simulink model "EncoderOffsetCalibrationF28069mLaunchPad"  (R2025b)
settings: Solver=FixedStepDiscrete  StartTime=0.0  StopTime=2  FixedStep=Ts  RelTol=1e-3  EnableMultiTasking=on
InitFcn:
  | OffsetCalibrationCallback;
  | motor.QEPSlits   = eval(get_param([bdroot '/Offset Calculation/Parameters/QEP Slits'], 'Value'));
  | target = mcb.getProcessorParameters('F28069M',PWM_frequency);
values from neighbouring files (symbols this model uses):
  PWM_frequency = eval(get_param([bdroot '/Open Loop Control/Parameters/PWM Frequency'], 'Value'))    [OpenloopMotorControlCallback.m]    (also in setup_offset_calculations.m = 20000)
  Ts = T_pwm    [OpenloopMotorControlCallback.m]    (also in setup_offset_calculations.m = 5e-05)
undefined symbols (not defined in the file or in its folder): bit, Down, GPTRIP1SEL, GPTRIP2SEL, TZ1, TZ2, Up
libraries: c2802xlib x4, simulink x3, mcbcontrolslib x3, c280xlib x3, svdschedulerlib x2, c2806xlib x2, mcbpositiondecoderlib x2, mcbeeMathTransformLib x1

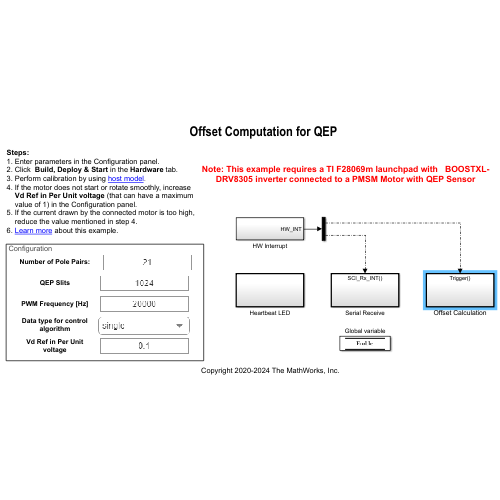
[thumbnail: Simulink's stored preview of the top-level diagram]
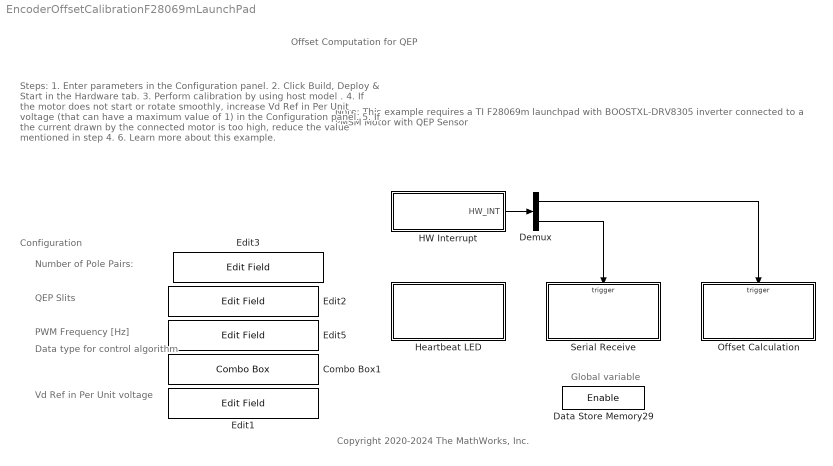
== system EncoderOffsetCalibrationF28069mLaunchPad ==
  note: Global variable
  note: Offset Computation for QEP
  note: Copyright 2020-2024 The MathWorks, Inc.
  note: QEP Slits
  note: PWM Frequency [Hz]
  note: Configuration
  note: Number of Pole Pairs:
  note: Data type for control algorithm
  note: Note: This example requires a TI F28069m launchpad with BOOSTXL-DRV8305 inverter connected to a PMSM Motor with QEP Sensor
  note: Steps:
      | 1. Enter parameters in the Configuration panel.
      | 2. Click Build, Deploy & Start in the Hardware tab.
      | 3. Perform calibration by using host model .
      | 4. If the motor does not start or rotate smoothly, increase
      | Vd Ref in Per Unit voltage (that can have a maximum
      | value of 1) in the Configuration panel.
      | 5. If the current drawn by the connected motor is too high,
      | reduce the value mentioned in step 4.
      | 6. Learn more about this example.
  note: Vd Ref in Per Unit voltage
  Combo Box1 : ComboBox  LabelPosition=Hide  SelectedLabel=single
  Data Store Memory29 : DataStoreMemory  DataStoreName=Enable  ReadBeforeWriteMsg=warning  WriteAfterWriteMsg=warning  WriteAfterReadMsg=warning  ShowAdditionalParam=off  OutDataTypeStr=boolean
  Demux : Demux  Outputs=2
  Edit{1..3,5} (4 alike) : EditField  LabelPosition=Hide  ShowInitialText=on  Alignment=Center
  HW Interrupt : Subsystem
  Heartbeat LED : Subsystem  TreatAsAtomicUnit=on
  Offset Calculation : Subsystem
  Serial Receive : Subsystem  SystemSampleTime=1e-3
  wires:
  HW Interrupt/1(HW_INT) -> Demux/1
  Demux/2 -> Serial Receive/Trigger
  Demux/1 -> Offset Calculation/Trigger

== system EncoderOffsetCalibrationF28069mLaunchPad/HW Interrupt ==
  HWI_ADCINT1 : svdschedulerlib/Hardware Interrupt v2  ISRGroup=ADC - Analog to Digital Converter  ISRName=ADCA1_INT  ISRNumber=32  NumEventsToServe=1  EventsList={'on','EOC event','1';'off','Overflow event','2';'off','Custom event','3'}  SelectedEvents={'event1'}  TaskPriority=30  DisablePreemption=off  ClearInterruptFlagsAtEndOfEvent=on  InterruptDefinitionFile=$(TARGET_ROOT)/registry/interrupts/F2837xS_interrupts.xml  HardwareBoard=F2837x  EnableSimPort=off
  HWI_SCIRXINTA : svdschedulerlib/Hardware Interrupt v2  ISRGroup=ADC - Analog to Digital Converter  ISRName=ADCA1_INT  ISRNumber=32  NumEventsToServe=1  EventsList={'on','EOC event','1';'off','Overflow event','2';'off','Custom event','3'}  SelectedEvents={'event1'}  TaskPriority=50  DisablePreemption=on  ClearInterruptFlagsAtEndOfEvent=on  InterruptDefinitionFile=$(TARGET_ROOT)/registry/interrupts/F2837xS_interrupts.xml  HardwareBoard=F2837x  EnableSimPort=off
  Mux : Mux  Inputs=2
  HW_INT : Outport
  wires:
  Mux/1 -> HW_INT/1
  HWI_ADCINT1/1 -> Mux/1
  HWI_SCIRXINTA/1 -> Mux/2

== system EncoderOffsetCalibrationF28069mLaunchPad/Heartbeat LED ==
  Digital Output1 : c2806xlib/Digital Output  GPIO_Number=GPIO32~GPIO39  GPIO_Bit0=off  GPIO_BIT0_Toggle=off  GPIO_Bit1=off  GPIO_BIT1_Toggle=off  GPIO_Bit2=on  GPIO_BIT2_Toggle=on  GPIO_Bit3=off  GPIO_BIT3_Toggle=off  GPIO_Bit4=off  GPIO_BIT4_Toggle=off  GPIO_Bit5=off  GPIO_BIT5_Toggle=off  GPIO_Bit6=off  GPIO_BIT6_Toggle=off  GPIO_Bit7=off  GPIO_BIT7_Toggle=off
  LED 1 Hz : Constant  OutDataTypeStr=uint16  SampleTime=0.5
  wires:
  LED 1 Hz/1 -> Digital Output1/1

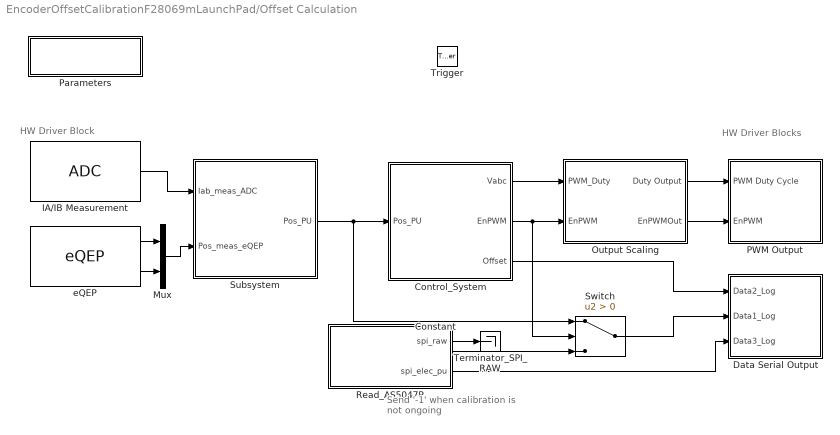
== system EncoderOffsetCalibrationF28069mLaunchPad/Offset Calculation ==
  note: HW Driver Blocks
  note: HW Driver Block
  note: Send '-1' when calibration is not ongoing
  Trigger : TriggerPort  TriggerType=function-call  VariantControl=Variant  PortDimensions=1
  Constant : Constant  Value=-1  OutDataTypeStr=dataType
  Control_System : Subsystem
  Data Serial Output : Subsystem
  IA/IB Measurement : c2802xlib/ADC  blkParamProc=C2000  ADCModule=1  samplingMode=Simultaneous sample mode  ADCResolution=12-bit (Single-ended input)  ADC29xResolution=12-bit  ADCMode=Single-ended input  useSOC1=SOC0  useSOC2=SOC0_SOC1  SOCAcquisitionWindow=7  SOCTriggerSource=ePWM4_ADCSOCA  SOCInterruptTrigger=No ADCINT  Ts=-1  dType=uint16  postInterrupt=on  interruptSel=ADCINT1  ADCINTContinuous=on  endma=off  chdma=1  conv1=ADCINA0  conv2=ADCINA3 and ADCINB3  conv1_Type4=ADCIN0  conv2_Type4=ADCIN0 and ADCIN1
  Mux : Mux  Inputs=2
  Output Scaling : Subsystem
  PWM Output : Subsystem
  Parameters : Subsystem
  Read_AS5047P : MATLAB Function  TreatAsAtomicUnit=on
  Subsystem : Subsystem
  Switch : Switch  Criteria=u2 > Threshold  SaturateOnIntegerOverflow=off  InputSameDT=off
  Terminator_SPI_RAW : Terminator
  eQEP : c280xlib/eQEP  useModule=eQEP1  pcInputmode=Quadrature-count  externalClockrate=2x resolution: Count the rising/falling edge  swapPolarityselection=Clockwise  qdfOutputport=off  qapPolarityselection=off  qbpPolarityselection=off  qipPolarityselection=off  qspPolarityselection=off  igatePolarityselection=off  sampleTime=-1  pcOutputport=on  pcMaximumvalue=4*1024 - 1  indexInitializationcheck=off  indexInitializationevent=Falling edge  strobeInitializationcheck=off  strobeInitializationevent=Rising edge  softwareInitializationcheck=off  softwareInitializationsource=Set to init value at start up  softwareInitializationmode=on  pcInitialvalue=0  pcResetmode=Reset on the first index event  ieloutputport=on  indexEventlatch=Rising edge  seloutputport=off  strobeEventlatch=Rising edge  pcefOutputport=off  enableEqepcapture=off  qctmrOutputport=off  qcprdOutputport=off  captureTimerprescaler=128  upEventprescaler=128  overflowErrorflag=off  directionErrorflag=off  captureTimerposition=On position counter read  unitTimerperiod=100000000  captureTimerlatch=off  capturePeriodlatch=off  positionCounterlatch=off  soenPolarityselection=off  spselPolarityselection=Index pin is used for sync output  compareValuesource=Specify via dialog  shadowMode=Load on QPOSCNT=0  compareValue=4294967295  syncOutputwidth=1  polaritySyncoutput=Active high  watchdogEnable=off  watchdogTimer=65535  outport1Datatype=auto  outport2Datatype=auto  outport3Datatype=auto  outport4Datatype=auto  outport5Datatype=auto  outport6Datatype=auto  outport7Datatype=auto  outport8Datatype=auto  outport9Datatype=auto  outport10Datatype=auto  outport11Datatype=auto  outport12Datatype=auto  eqepinterrupt_pce=off  eqepinterrupt_qpe=off  eqepinterrupt_qdc=off  eqepinterrupt_wto=off  eqepinterrupt_pcu=off  eqepinterrupt_pco=off  eqepinterrupt_pcr=off  eqepinterrupt_pcm=off  eqepinterrupt_sel=off  eqepinterrupt_iel=off  eqepinterrupt_uto=off  pheOutputport=off  watchdogOutputport=off  outport13Datatype=auto  outport14Datatype=auto
  wires:
  Control_System/1(Vabc) -> Output Scaling/1(PWM_Duty)
  Output Scaling/1(Duty Output) -> PWM Output/1(PWM Duty Cycle)
  eQEP/1 -> Mux/1
  IA/IB Measurement/1 -> Subsystem/1(Iab_meas_ADC)
  eQEP/2 -> Mux/2
  Mux/1 -> Subsystem/2(Pos_meas_eQEP)
  Subsystem/1(Pos_PU) -> Switch/1, Control_System/1(Pos_PU)
  Control_System/3(Offset) -> Data Serial Output/1(Data2_Log)
  Control_System/2(EnPWM) -> Switch/2, Output Scaling/2(EnPWM)
  Output Scaling/2(EnPWMOut) -> PWM Output/2(EnPWM)
  Constant/1 -> Switch/3
  Switch/1 -> Data Serial Output/2(Data1_Log)
  Read_AS5047P/2(spi_elec_pu) -> Data Serial Output/3(Data3_Log)
  Read_AS5047P/1(spi_raw) -> Terminator_SPI_RAW/1

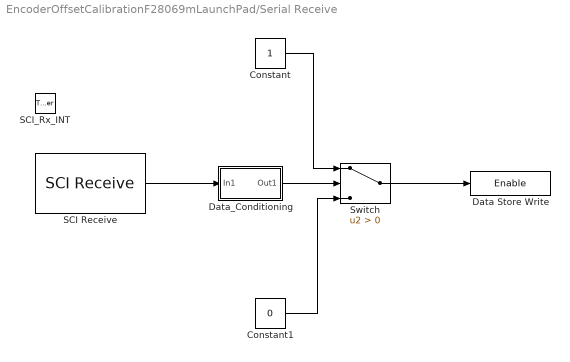
== system EncoderOffsetCalibrationF28069mLaunchPad/Serial Receive ==
  SCI_Rx_INT : TriggerPort  TriggerType=function-call  VariantControl=Variant
  Constant : Constant  OutDataTypeStr=boolean
  Constant1 : Constant  Value=0  OutDataTypeStr=boolean
  Data Store Write : DataStoreWrite  DataStoreName=Enable  IndexOptions=Index vector (dialog)  Indices=1  OutputSizes=1
  Data_Conditioning : Subsystem
  SCI Receive : c280xlib/SCI Receive  sciModule=A  dataHead=''  headerCheckMaxCount=16  dataTail=''  dataType=uint16  dataLenOptions=Length via dialog  dataDim=1  maxDataLength=1  initValue=0  errOption=Output custom value  errValue=0  sampleTime=-1  blockingMode=on  timeOut=0.019444  outputStatus=off
  Switch : Switch  Criteria=u2 > Threshold  SaturateOnIntegerOverflow=off  InputSameDT=off
  wires:
  SCI Receive/1 -> Data_Conditioning/1(In1)
  Data_Conditioning/1(Out1) -> Switch/2
  Switch/1 -> Data Store Write/1
  Constant/1 -> Switch/1
  Constant1/1 -> Switch/3

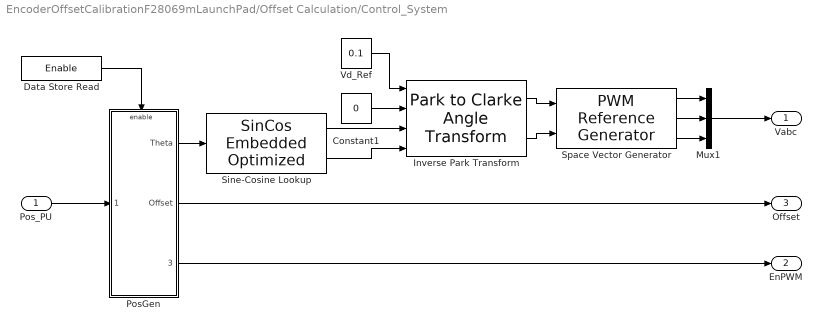
== system EncoderOffsetCalibrationF28069mLaunchPad/Offset Calculation/Control_System ==
  Pos_PU : Inport
  Constant1 : Constant  Value=0  OutDataTypeStr=dataType  SampleTime=-1
  Data Store Read : DataStoreRead  DataStoreName=Enable  IndexOptions=Index vector (dialog)  Indices=1  OutputSizes=1
  Inverse Park Transform : mcbeeMathTransformLib/Park to Clarke Angle Transform  AxisAlignment=D-axis  UseWithEmbedded=on  PhaseInput=Two inputs  ThetaInput=Sine and Cosine electrical position  AngleInput=Per-unit  N_points=1024
  Mux1 : Mux  Inputs=3
  PosGen : Subsystem
  Sine-Cosine Lookup : mcbcontrolslib/SinCos Embedded Optimized  LabelModeActiveChoice=MCB_Sin  OptforProc=off  ApproximationMethod=None  UserApproxMethod=Lookup  ApproxStatus=None  InterpMethod=Linear point-slope  NumberOfDataPoints=16  NumberOfIterations=11  RemoveProtectionAgainstOutOfRangeInput=off  TableDataTypeStr=Inherit: Inherit via input  AngleInput=Per-unit  ThetaDataType=single  N_points=1024  DatatypeInput=Inherit from input  Datatype=Inherit: Same as input
  Space Vector Generator : mcbcontrolslib/PWM Reference Generator  inSignal=Valphabeta  modType=SVM: space vector modulation
  Vd_Ref : Constant  Value=0.1  OutDataTypeStr=dataType  SampleTime=-1
  Vabc : Outport  VectorParamsAs1DForOutWhenUnconnected=off
  EnPWM : Outport  Port=2  VectorParamsAs1DForOutWhenUnconnected=off
  Offset : Outport  Port=3  VectorParamsAs1DForOutWhenUnconnected=off
  wires:
  PosGen/1(Theta) -> Sine-Cosine Lookup/1
  Sine-Cosine Lookup/1 -> Inverse Park Transform/3
  Space Vector Generator/2 -> Mux1/2
  Space Vector Generator/1 -> Mux1/1
  Inverse Park Transform/2 -> Space Vector Generator/2
  Inverse Park Transform/1 -> Space Vector Generator/1
  Sine-Cosine Lookup/2 -> Inverse Park Transform/4
  Space Vector Generator/3 -> Mux1/3
  Pos_PU/1 -> PosGen/1(Pos_In)
  Constant1/1 -> Inverse Park Transform/2
  Vd_Ref/1 -> Inverse Park Transform/1
  PosGen/2(Offset) -> Offset/1
  PosGen/3(EnPWM) -> EnPWM/1
  Data Store Read/1 -> PosGen/Enable
  Mux1/1 -> Vabc/1

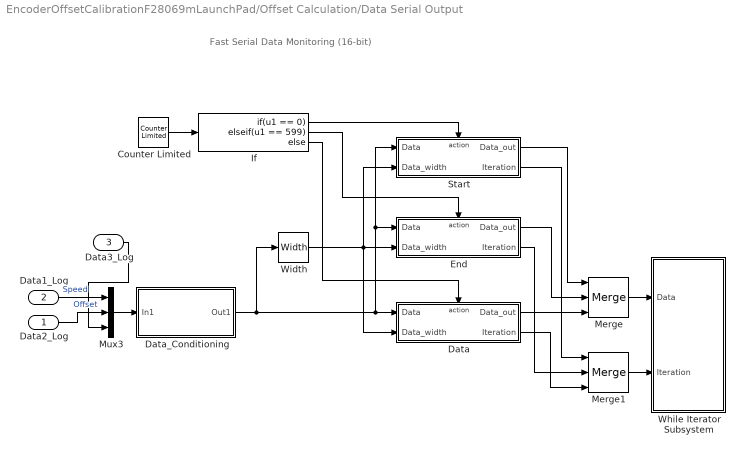
== system EncoderOffsetCalibrationF28069mLaunchPad/Offset Calculation/Data Serial Output ==
  note: Fast Serial Data Monitoring (16-bit)
  Data2_Log : Inport
  Data1_Log : Inport  Port=2
  Data3_Log : Inport  Port=3
  Counter Limited : simulink/Sources/Counter Limited  uplimit=599  tsamp=-1
  Data : Subsystem  TreatAsAtomicUnit=on
  Data_Conditioning : Subsystem
  End : Subsystem  TreatAsAtomicUnit=on
  If : If  IfExpression=u1 == 0  ElseIfExpressions=u1 == 599
  Merge : Merge  Inputs=3
  Merge1 : Merge  Inputs=3
  Mux3 : Mux  Inputs=3
  Start : Subsystem  TreatAsAtomicUnit=on
  While Iterator Subsystem : Subsystem  TreatAsAtomicUnit=on
  Width : Width  OutDataTypeMode=All ports same datatype  DataType=uint16
  wires:
  Merge/1 -> While Iterator Subsystem/1(Data)
  If/2 -> End/Action
  If/3 -> Data/Action
  Counter Limited/1 -> If/1
  End/1(Data_out) -> Merge/2
  Width/1 -> Data/2(Data_width), Start/2(Data_width), End/2(Data_width)
  Start/1(Data_out) -> Merge/1
  Start/2(Iteration) -> Merge1/1
  Merge1/1 -> While Iterator Subsystem/2(Iteration)
  Data/1(Data_out) -> Merge/3
  If/1 -> Start/Action
  End/2(Iteration) -> Merge1/2
  Data/2(Iteration) -> Merge1/3
  Data2_Log/1 -> Mux3/2  "Offset"
  Data1_Log/1 -> Mux3/1  "Speed"
  Data_Conditioning/1(Out1) -> Width/1, Start/1(Data), End/1(Data), Data/1(Data)
  Mux3/1 -> Data_Conditioning/1(In1)
  Data3_Log/1 -> Mux3/3

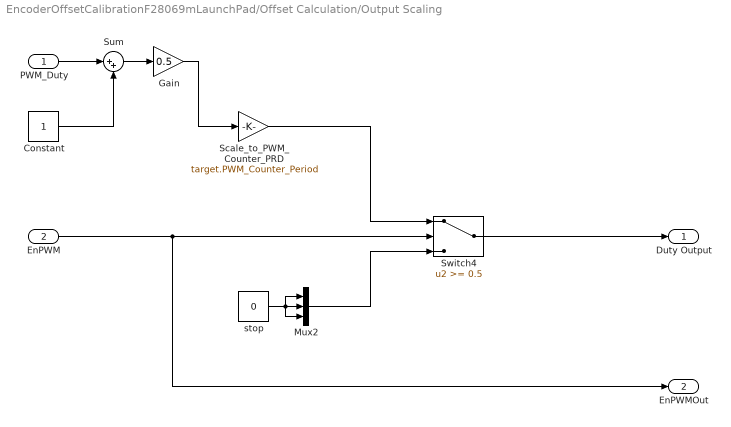
== system EncoderOffsetCalibrationF28069mLaunchPad/Offset Calculation/Output Scaling ==
  PWM_Duty : Inport
  EnPWM : Inport  Port=2
  Constant : Constant  OutDataTypeStr=Inherit: Inherit via back propagation
  Gain : Gain  Gain=0.5  OutDataTypeStr=Inherit: Same as input
  Mux2 : Mux  Inputs=3
  Scale_to_PWM_Counter_PRD : Gain  Gain=target.PWM_Counter_Period  OutDataTypeStr=uint16  RndMeth=Simplest
  Sum : Sum  Inputs=|++
  Switch4 : Switch  Threshold=0.5  SaturateOnIntegerOverflow=off  InputSameDT=off
  stop : Constant  Value=0  OutDataTypeStr=uint16
  Duty Output : Outport
  EnPWMOut : Outport  Port=2
  wires:
  PWM_Duty/1 -> Sum/1
  stop/1 -> Mux2/3, Mux2/2, Mux2/1
  Switch4/1 -> Duty Output/1
  Sum/1 -> Gain/1
  Constant/1 -> Sum/2
  Mux2/1 -> Switch4/3
  Gain/1 -> Scale_to_PWM_Counter_PRD/1
  Scale_to_PWM_Counter_PRD/1 -> Switch4/1
  EnPWM/1 -> EnPWMOut/1, Switch4/2

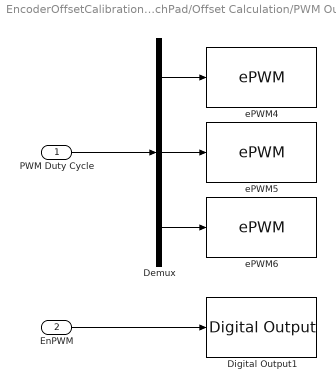
== system EncoderOffsetCalibrationF28069mLaunchPad/Offset Calculation/PWM Output ==
  PWM Duty Cycle : Inport
  EnPWM : Inport  Port=2
  Demux : Demux  Outputs=3
  Digital Output1 : c2806xlib/Digital Output  GPIO_Number=GPIO50~GPIO55  GPIO_Bit0=off  GPIO_BIT0_Toggle=off  GPIO_Bit1=off  GPIO_BIT1_Toggle=off  GPIO_Bit2=on  GPIO_BIT2_Toggle=off  GPIO_Bit3=off  GPIO_BIT3_Toggle=off  GPIO_Bit4=off  GPIO_BIT4_Toggle=off  GPIO_Bit5=off  GPIO_BIT5_Toggle=off  GPIO_Bit6=off  GPIO_BIT6_Toggle=off  GPIO_Bit7=off  GPIO_BIT7_Toggle=off
  ePWM4 : c2802xlib/ePWM  PwmType=C2000  useModule=ePWM4  ePWMxLINKTBPRD=Not Linked  periodUnits=Clock cycles  timerSource=Specify via dialog  timerPeriod_clk=target.PWM_Counter_Period  timerPeriod_sec=64000  tbshadow=Counter equals to zero  countingMode=Up-Down  phaseActiveEnable=Disable  phaseDirection=Count down after sync  phaseActive=0  synchronizationEnable=off  dcaevt1Sync=off  dcbevt1Sync=off  synchronizationOption=Counter equals to zero (CTR=Zero)  dcbevt1SyncOut=off  dcaevt1SyncOut=off  cmpdSyncOut=off  cmpcSyncOut=off  cmpbSyncOut=off  zeroSyncOut=on  swfSyncOut=off  perSynchronizationOption=Counter equals to period (CTR=PRD)  clockPrescale=1  HSclockPrescale=1  enswap=off  ePWMxAStatus=on  ePWMxAactionLogic1=Do nothing  ePWMxAactionLogic2=Do nothing  ePWMxAactionLogic3=Clear  ePWMxAactionLogic4=Set  ePWMxAactionLogic5=Do nothing  ePWMxAactionLogic6=Do nothing  ePWMxACSFenable=off  ePWMxACSFvalue=Forcing disable  ePWMxASFreload=Zero  ePWMxBStatus=off  ePWMxBactionLogic1=Do nothing  ePWMxBactionLogic2=Set  ePWMxBactionLogic3=Do nothing  ePWMxBactionLogic4=Do nothing  ePWMxBactionLogic5=Clear  ePWMxBactionLogic6=Do nothing  ePWMxBCSFenable=off  ePWMxBCSFvalue=Forcing disable  ePWMxBSFreload=Zero  ePWNxBOutWay=off  ePWMxLINKCMPA=Not Linked  CMPAUnits=Clock cycles  CMPASource=Input port  CMPAValue_per=32000  CMPAValue_clk=floor(target.PWM_Counter_Period/2+1)  enCMPAshadow=Counter equals to zero (CTR=Zero)  ePWMxLINKCMPB=Not Linked  CMPBUnits=Clock cycles  CMPBSource=Specify via dialog  CMPBValue_per=50  CMPBValue_clk=floor(target.PWM_Counter_Period/2+1)  enCMPBshadow=Counter equals to zero (CTR=Zero)  ePWMxLINKCMPC=Not Linked  CMPCUnits=Clock cycles  CMPCSource=Specify via dialog  CMPCValue_per=50  CMPCValue_clk=32000  enCMPCshadow=Counter equals to zero (CTR=Zero)  ePWMxLINKCMPD=Not Linked  CMPDUnits=Clock cycles  CMPDSource=Specify via dialog  CMPDValue_per=50  CMPDValue_clk=32000  enCMPDshadow=Counter equals to zero (CTR=Zero)  enableDBePWMxA=on  enableDBePWMxB=on  enhalfcycle=off  DBpolarity=Active high complementary (AHC)  DBedgeDelay=Positive  DBSource_ePWMxA=ePWMxA  DBSource_ePWMxB=ePWMxA  DBPeriodUnits=Clock cycles  DBperiodSource=Specify via dialog  REDperiod=5  FEDperiod=5  REDperiod_sec=0  FEDperiod_sec=0  LoadModeDBRED=Immediate without using shadow  LoadModeDBFED=Immediate without using shadow  adcstartModuleA=on  adcrequestEventA=First event  adcstartEventA=Counter equals to period (CTR=PRD)  adcstartEventA_type2=Digital Compare Module A Event 1 start of conversion (DCAEVT1.soc)  adcstartModuleB=off  adcrequestEventB=First event  adcstartEventB=Counter equals to zero (CTR=Zero)  adcstartEventB_type2=Counter equals to zero (CTR=Zero)  intEn=off  intPrd=First event  intSel=Counter equals to zero (CTR=Zero)  intSel_type2=Counter equals to zero (CTR=Zero)  hrpe=off  enHRPWM=off  HRPWM_LoadMode=Counter equals to period (CTR=PRD)  HRPWM_CTLMode=Duty or Period control mode  HRPWM_EDGMode=Both edge  hrpeb=off  enHRPWMB=off  HRPWM_LoadModeB=Counter equals to zero (CTR=ZERO)  HRPWM_CTLModeB=Duty or Period control mode  HRPWM_EDGModeB=Both edge  enHRDBRED=off  enHRDBFED=off  enSFO=on  enautoconv=on  chopperEnable=off  chopperFrequency=1  chopperFirstwidth=1  chopperDuty=12.5%  tripZonesource=Specify via dialog  tzselOSHT1=off  tzselOSHT2=off  tzselOSHT3=off  tzselOSHT4=off  tzselOSHT5=off  tzselOSHT6=off  tzselOSHDCAEV1=off  tzselOSHDCBEV1=off  tzselCBC1=off  tzselCBC2=off  tzselCBC3=off  tzselCBC4=off  tzselCBC5=off  tzselCBC6=off  tzselCBCDCAEV2=off  tzselCBCDCBEV2=off  enTzOstIntr=off  enTzCbcIntr=off  enTzDCAEVT1Intr=off  enTzDCAEVT2Intr=off  enTzDCBEVT1Intr=off  enTzDCBEVT2Intr=off  tzclrCBCLatch=Counter equals to zero (CTR=Zero)  ePWMxAforced=No action  ePWMxBforced=No action  DCAEVT1forced=No action  DCBEVT1forced=No action  DCAEVT2forced=No action  DCBEVT2forced=No action  dcah=Trip Zone 1 input (TZ1)  dcal=Trip Zone 2 input (TZ2)  dcbh=Trip Zone 1 input (TZ1)  dcbl=Trip Zone 2 input (TZ2)  dcah_type2=GPTRIP1SEL/(TZ1)  dcal_type2=GPTRIP2SEL/(TZ2)  dcbh_type2=GPTRIP1SEL/(TZ1)  dcbl_type2=GPTRIP2SEL/(TZ2)  gendcaevt1=Event disabled  gendcaevt2=Event disabled  gendcbevt1=Event disabled  gendcbevt2=Event disabled  dcaevt1src=DCAEVT1 with sync  dcaevt2src=DCAEVT2 with sync  dcbevt1src=DCBEVT1 with sync  dcbevt2src=DCBEVT2 with sync  pulsesel=Counter equals to zero (CTR=Zero)  blankinv=off  blankoffset=0  blankwidth=0  evsrcsel=Filtered version of DCAEVT1 (DCAEVT1FILT)  encape=off
  ePWM5 : c2802xlib/ePWM  PwmType=C2000  useModule=ePWM5  ePWMxLINKTBPRD=Not Linked  periodUnits=Clock cycles  timerSource=Specify via dialog  timerPeriod_clk=target.PWM_Counter_Period  timerPeriod_sec=64000  tbshadow=Counter equals to zero  countingMode=Up-Down  phaseActiveEnable=Set counter to phase value specified via dialog  phaseDirection=Count up after sync  phaseActive=0  synchronizationEnable=off  dcaevt1Sync=off  dcbevt1Sync=off  synchronizationOption=Pass through (EPWMxSYNCI or SWFSYNC)  dcbevt1SyncOut=off  dcaevt1SyncOut=off  cmpdSyncOut=off  cmpcSyncOut=off  cmpbSyncOut=off  zeroSyncOut=off  swfSyncOut=on  perSynchronizationOption=Counter equals to period (CTR=PRD)  clockPrescale=1  HSclockPrescale=1  enswap=off  ePWMxAStatus=on  ePWMxAactionLogic1=Do nothing  ePWMxAactionLogic2=Do nothing  ePWMxAactionLogic3=Clear  ePWMxAactionLogic4=Set  ePWMxAactionLogic5=Do nothing  ePWMxAactionLogic6=Do nothing  ePWMxACSFenable=off  ePWMxACSFvalue=Forcing disable  ePWMxASFreload=Zero  ePWMxBStatus=off  ePWMxBactionLogic1=Do nothing  ePWMxBactionLogic2=Set  ePWMxBactionLogic3=Do nothing  ePWMxBactionLogic4=Do nothing  ePWMxBactionLogic5=Clear  ePWMxBactionLogic6=Do nothing  ePWMxBCSFenable=off  ePWMxBCSFvalue=Forcing disable  ePWMxBSFreload=Zero  ePWNxBOutWay=off  ePWMxLINKCMPA=Not Linked  CMPAUnits=Clock cycles  CMPASource=Input port  CMPAValue_per=32000  CMPAValue_clk=floor(target.PWM_Counter_Period/2+1)  enCMPAshadow=Counter equals to zero (CTR=Zero)  ePWMxLINKCMPB=Not Linked  CMPBUnits=Clock cycles  CMPBSource=Specify via dialog  CMPBValue_per=50  CMPBValue_clk=floor(target.PWM_Counter_Period/2+1)  enCMPBshadow=Counter equals to zero (CTR=Zero)  ePWMxLINKCMPC=Not Linked  CMPCUnits=Clock cycles  CMPCSource=Specify via dialog  CMPCValue_per=50  CMPCValue_clk=32000  enCMPCshadow=Counter equals to zero (CTR=Zero)  ePWMxLINKCMPD=Not Linked  CMPDUnits=Clock cycles  CMPDSource=Specify via dialog  CMPDValue_per=50  CMPDValue_clk=32000  enCMPDshadow=Counter equals to zero (CTR=Zero)  enableDBePWMxA=on  enableDBePWMxB=on  enhalfcycle=off  DBpolarity=Active high complementary (AHC)  DBedgeDelay=Positive  DBSource_ePWMxA=ePWMxA  DBSource_ePWMxB=ePWMxA  DBPeriodUnits=Clock cycles  DBperiodSource=Specify via dialog  REDperiod=5  FEDperiod=5  REDperiod_sec=0  FEDperiod_sec=0  LoadModeDBRED=Immediate without using shadow  LoadModeDBFED=Immediate without using shadow  adcstartModuleA=off  adcrequestEventA=First event  adcstartEventA=Digital Compare Module A Event 1 start of conversion (DCAEVT1.soc)  adcstartEventA_type2=Digital Compare Module A Event 1 start of conversion (DCAEVT1.soc)  adcstartModuleB=off  adcrequestEventB=First event  adcstartEventB=Counter equals to zero (CTR=Zero)  adcstartEventB_type2=Counter equals to zero (CTR=Zero)  intEn=off  intPrd=First event  intSel=Counter equals to zero (CTR=Zero)  intSel_type2=Counter equals to zero (CTR=Zero)  hrpe=off  enHRPWM=off  HRPWM_LoadMode=Counter equals to period (CTR=PRD)  HRPWM_CTLMode=Duty or Period control mode  HRPWM_EDGMode=Both edge  hrpeb=off  enHRPWMB=off  HRPWM_LoadModeB=Counter equals to zero (CTR=ZERO)  HRPWM_CTLModeB=Duty or Period control mode  HRPWM_EDGModeB=Both edge  enHRDBRED=off  enHRDBFED=off  enSFO=on  enautoconv=on  chopperEnable=off  chopperFrequency=1  chopperFirstwidth=1  chopperDuty=12.5%  tripZonesource=Specify via dialog  tzselOSHT1=off  tzselOSHT2=off  tzselOSHT3=off  tzselOSHT4=off  tzselOSHT5=off  tzselOSHT6=off  tzselOSHDCAEV1=off  tzselOSHDCBEV1=off  tzselCBC1=off  tzselCBC2=off  tzselCBC3=off  tzselCBC4=off  tzselCBC5=off  tzselCBC6=off  tzselCBCDCAEV2=off  tzselCBCDCBEV2=off  enTzOstIntr=off  enTzCbcIntr=off  enTzDCAEVT1Intr=off  enTzDCAEVT2Intr=off  enTzDCBEVT1Intr=off  enTzDCBEVT2Intr=off  tzclrCBCLatch=Counter equals to zero (CTR=Zero)  ePWMxAforced=No action  ePWMxBforced=No action  DCAEVT1forced=No action  DCBEVT1forced=No action  DCAEVT2forced=No action  DCBEVT2forced=No action  dcah=Trip Zone 1 input (TZ1)  dcal=Trip Zone 2 input (TZ2)  dcbh=Trip Zone 1 input (TZ1)  dcbl=Trip Zone 2 input (TZ2)  dcah_type2=GPTRIP1SEL/(TZ1)  dcal_type2=GPTRIP2SEL/(TZ2)  dcbh_type2=GPTRIP1SEL/(TZ1)  dcbl_type2=GPTRIP2SEL/(TZ2)  gendcaevt1=Event disabled  gendcaevt2=Event disabled  gendcbevt1=Event disabled  gendcbevt2=Event disabled  dcaevt1src=DCAEVT1 with sync  dcaevt2src=DCAEVT2 with sync  dcbevt1src=DCBEVT1 with sync  dcbevt2src=DCBEVT2 with sync  pulsesel=Counter equals to zero (CTR=Zero)  blankinv=off  blankoffset=0  blankwidth=0  evsrcsel=Filtered version of DCAEVT1 (DCAEVT1FILT)  encape=off
  ePWM6 : c2802xlib/ePWM  PwmType=C2000  useModule=ePWM6  ePWMxLINKTBPRD=Not Linked  periodUnits=Clock cycles  timerSource=Specify via dialog  timerPeriod_clk=target.PWM_Counter_Period  timerPeriod_sec=64000  tbshadow=Counter equals to zero  countingMode=Up-Down  phaseActiveEnable=Set counter to phase value specified via dialog  phaseDirection=Count up after sync  phaseActive=0  synchronizationEnable=off  dcaevt1Sync=off  dcbevt1Sync=off  synchronizationOption=Disable  dcbevt1SyncOut=off  dcaevt1SyncOut=off  cmpdSyncOut=off  cmpcSyncOut=off  cmpbSyncOut=off  zeroSyncOut=off  swfSyncOut=off  perSynchronizationOption=Counter equals to period (CTR=PRD)  clockPrescale=1  HSclockPrescale=1  enswap=off  ePWMxAStatus=on  ePWMxAactionLogic1=Do nothing  ePWMxAactionLogic2=Do nothing  ePWMxAactionLogic3=Clear  ePWMxAactionLogic4=Set  ePWMxAactionLogic5=Do nothing  ePWMxAactionLogic6=Do nothing  ePWMxACSFenable=off  ePWMxACSFvalue=Forcing disable  ePWMxASFreload=Zero  ePWMxBStatus=off  ePWMxBactionLogic1=Do nothing  ePWMxBactionLogic2=Set  ePWMxBactionLogic3=Do nothing  ePWMxBactionLogic4=Do nothing  ePWMxBactionLogic5=Clear  ePWMxBactionLogic6=Do nothing  ePWMxBCSFenable=off  ePWMxBCSFvalue=Forcing disable  ePWMxBSFreload=Zero  ePWNxBOutWay=off  ePWMxLINKCMPA=Not Linked  CMPAUnits=Clock cycles  CMPASource=Input port  CMPAValue_per=32000  CMPAValue_clk=floor(target.PWM_Counter_Period/2+1)  enCMPAshadow=Counter equals to zero (CTR=Zero)  ePWMxLINKCMPB=Not Linked  CMPBUnits=Clock cycles  CMPBSource=Specify via dialog  CMPBValue_per=50  CMPBValue_clk=floor(target.PWM_Counter_Period/2+1)  enCMPBshadow=Counter equals to zero (CTR=Zero)  ePWMxLINKCMPC=Not Linked  CMPCUnits=Clock cycles  CMPCSource=Specify via dialog  CMPCValue_per=50  CMPCValue_clk=32000  enCMPCshadow=Counter equals to zero (CTR=Zero)  ePWMxLINKCMPD=Not Linked  CMPDUnits=Clock cycles  CMPDSource=Specify via dialog  CMPDValue_per=50  CMPDValue_clk=32000  enCMPDshadow=Counter equals to zero (CTR=Zero)  enableDBePWMxA=on  enableDBePWMxB=on  enhalfcycle=off  DBpolarity=Active high complementary (AHC)  DBedgeDelay=Positive  DBSource_ePWMxA=ePWMxA  DBSource_ePWMxB=ePWMxA  DBPeriodUnits=Clock cycles  DBperiodSource=Specify via dialog  REDperiod=5  FEDperiod=5  REDperiod_sec=0  FEDperiod_sec=0  LoadModeDBRED=Immediate without using shadow  LoadModeDBFED=Immediate without using shadow  adcstartModuleA=off  adcrequestEventA=First event  adcstartEventA=Digital Compare Module A Event 1 start of conversion (DCAEVT1.soc)  adcstartEventA_type2=Digital Compare Module A Event 1 start of conversion (DCAEVT1.soc)  adcstartModuleB=off  adcrequestEventB=First event  adcstartEventB=Counter equals to zero (CTR=Zero)  adcstartEventB_type2=Counter equals to zero (CTR=Zero)  intEn=off  intPrd=First event  intSel=Counter equals to zero (CTR=Zero)  intSel_type2=Counter equals to zero (CTR=Zero)  hrpe=off  enHRPWM=off  HRPWM_LoadMode=Counter equals to period (CTR=PRD)  HRPWM_CTLMode=Duty or Period control mode  HRPWM_EDGMode=Both edge  hrpeb=off  enHRPWMB=off  HRPWM_LoadModeB=Counter equals to zero (CTR=ZERO)  HRPWM_CTLModeB=Duty or Period control mode  HRPWM_EDGModeB=Both edge  enHRDBRED=off  enHRDBFED=off  enSFO=on  enautoconv=on  chopperEnable=off  chopperFrequency=1  chopperFirstwidth=1  chopperDuty=12.5%  tripZonesource=Specify via dialog  tzselOSHT1=off  tzselOSHT2=off  tzselOSHT3=off  tzselOSHT4=off  tzselOSHT5=off  tzselOSHT6=off  tzselOSHDCAEV1=off  tzselOSHDCBEV1=off  tzselCBC1=off  tzselCBC2=off  tzselCBC3=off  tzselCBC4=off  tzselCBC5=off  tzselCBC6=off  tzselCBCDCAEV2=off  tzselCBCDCBEV2=off  enTzOstIntr=off  enTzCbcIntr=off  enTzDCAEVT1Intr=off  enTzDCAEVT2Intr=off  enTzDCBEVT1Intr=off  enTzDCBEVT2Intr=off  tzclrCBCLatch=Counter equals to zero (CTR=Zero)  ePWMxAforced=No action  ePWMxBforced=No action  DCAEVT1forced=No action  DCBEVT1forced=No action  DCAEVT2forced=No action  DCBEVT2forced=No action  dcah=Trip Zone 1 input (TZ1)  dcal=Trip Zone 2 input (TZ2)  dcbh=Trip Zone 1 input (TZ1)  dcbl=Trip Zone 2 input (TZ2)  dcah_type2=GPTRIP1SEL/(TZ1)  dcal_type2=GPTRIP2SEL/(TZ2)  dcbh_type2=GPTRIP1SEL/(TZ1)  dcbl_type2=GPTRIP2SEL/(TZ2)  gendcaevt1=Event disabled  gendcaevt2=Event disabled  gendcbevt1=Event disabled  gendcbevt2=Event disabled  dcaevt1src=DCAEVT1 with sync  dcaevt2src=DCAEVT2 with sync  dcbevt1src=DCBEVT1 with sync  dcbevt2src=DCBEVT2 with sync  pulsesel=Counter equals to zero (CTR=Zero)  blankinv=off  blankoffset=0  blankwidth=0  evsrcsel=Filtered version of DCAEVT1 (DCAEVT1FILT)  encape=off
  wires:
  Demux/1 -> ePWM4/1
  Demux/2 -> ePWM5/1
  PWM Duty Cycle/1 -> Demux/1
  Demux/3 -> ePWM6/1
  EnPWM/1 -> Digital Output1/1

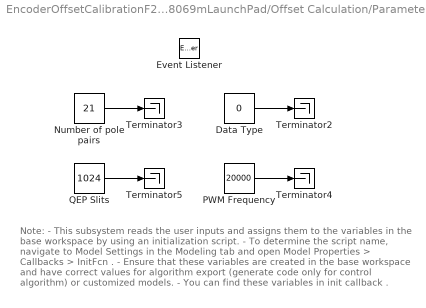
== system EncoderOffsetCalibrationF28069mLaunchPad/Offset Calculation/Parameters ==
  note: Note:
      | - This subsystem reads the user inputs and assigns them to the
      | variables in the base workspace by using an initialization script.
      | - To determine the script name, navigate to Model Settings in the
      | Modeling tab and open Model Properties > Callbacks >
      | InitFcn .
      | - Ensure that these variables are created in the base workspace
      | and have correct values for algorithm export (generate code
      | only for control algorithm) or customized models.
      | - You can find these variables in init callback .
  Data Type : Constant  Value=0
  Event Listener : EventListener  DisableCoverage=on  EventName=reset
  Number of pole pairs : Constant  Value=21
  PWM Frequency : Constant  Value=20000
  QEP Slits : Constant  Value=1024
  Terminator{2..5} (4 alike) : Terminator
  wires:
  Data Type/1 -> Terminator2/1
  Number of pole pairs/1 -> Terminator3/1
  PWM Frequency/1 -> Terminator4/1
  QEP Slits/1 -> Terminator5/1

== system EncoderOffsetCalibrationF28069mLaunchPad/Offset Calculation/Subsystem ==
  Iab_meas_ADC : Inport
  Pos_meas_eQEP : Inport  Port=2
  "Calculate Position from QEP count " : Subsystem
  Demux : Demux  Outputs=2
  Terminator : Terminator
  Pos_PU : Outport  InitialOutput=0  VectorParamsAs1DForOutWhenUnconnected=off
  wires:
  "Calculate Position from QEP count "/1(Theta_e) -> Pos_PU/1
  Demux/2 -> "Calculate Position from QEP count "/2(Index)
  Pos_meas_eQEP/1 -> Demux/1
  Demux/1 -> "Calculate Position from QEP count "/1(Count)
  Iab_meas_ADC/1 -> Terminator/1

== system EncoderOffsetCalibrationF28069mLaunchPad/Serial Receive/Data_Conditioning ==
  In1 : Inport
  Data Type Conversion1 : DataTypeConversion  OutDataTypeStr=dataType  RndMeth=Simplest  SaturateOnIntegerOverflow=off
  Data Type Conversion2 : DataTypeConversion  OutDataTypeStr=uint16  ConvertRealWorld=Stored Integer (SI)  RndMeth=Simplest  SaturateOnIntegerOverflow=off
  Out1 : Outport  VectorParamsAs1DForOutWhenUnconnected=off
  wires:
  Data Type Conversion1/1 -> Out1/1
  In1/1 -> Data Type Conversion2/1
  Data Type Conversion2/1 -> Data Type Conversion1/1

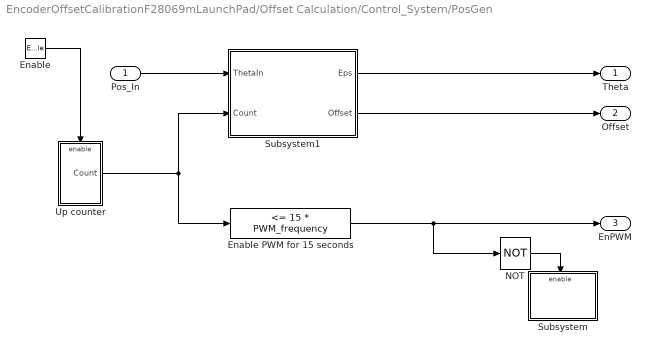
== system EncoderOffsetCalibrationF28069mLaunchPad/Offset Calculation/Control_System/PosGen ==
  Pos_In : Inport
  Enable : EnablePort  StatesWhenEnabling=reset  ShowOutputPort=on
  Enable PWM for 15 seconds : simulink/Logic and Bit Operations/Compare To Constant  relop=<=  const=15 * PWM_frequency  OutDataTypeStr=boolean
  NOT : Logic  Operator=NOT  IconShape=distinctive  AllPortsSameDT=off  OutDataTypeStr=boolean
  Subsystem : Subsystem
  Subsystem1 : Subsystem
  Up counter : Subsystem
  Theta : Outport
  Offset : Outport  Port=2
  EnPWM : Outport  Port=3  OutputWhenDisabled=reset  InitialOutput=0
  wires:
  Subsystem1/1(Eps) -> Theta/1
  Pos_In/1 -> Subsystem1/1(ThetaIn)
  Up counter/1(Count) -> Enable PWM for 15 seconds/1, Subsystem1/2(Count)
  Enable/1 -> Up counter/Enable
  Enable PWM for 15 seconds/1 -> NOT/1, EnPWM/1
  NOT/1 -> Subsystem/Enable
  Subsystem1/2(Offset) -> Offset/1

== system EncoderOffsetCalibrationF28069mLaunchPad/Offset Calculation/Data Serial Output/Data ==
  Data : Inport
  Data_width : Inport  Port=2
  Action Port : ActionPort  ActionPortLabel=else
  Mux : Mux  Inputs=2
  Start : Constant  Value=hex2dec('0000')  OutDataTypeStr=uint16
  Data_out : Outport  VectorParamsAs1DForOutWhenUnconnected=off
  Iteration : Outport  Port=2  VectorParamsAs1DForOutWhenUnconnected=off
  wires:
  Start/1 -> Mux/2
  Mux/1 -> Data_out/1
  Data/1 -> Mux/1
  Data_width/1 -> Iteration/1

== system EncoderOffsetCalibrationF28069mLaunchPad/Offset Calculation/Data Serial Output/Data_Conditioning ==
  In1 : Inport
  Data Type Conversion1 : DataTypeConversion  OutDataTypeStr=fixdt(1,32,12)  RndMeth=Simplest  SaturateOnIntegerOverflow=off
  Data Type Conversion3 : DataTypeConversion  OutDataTypeStr=uint16  ConvertRealWorld=Stored Integer (SI)  SaturateOnIntegerOverflow=off  RndMeth=Floor
  Out1 : Outport
  wires:
  Data Type Conversion1/1 -> Data Type Conversion3/1
  Data Type Conversion3/1 -> Out1/1
  In1/1 -> Data Type Conversion1/1

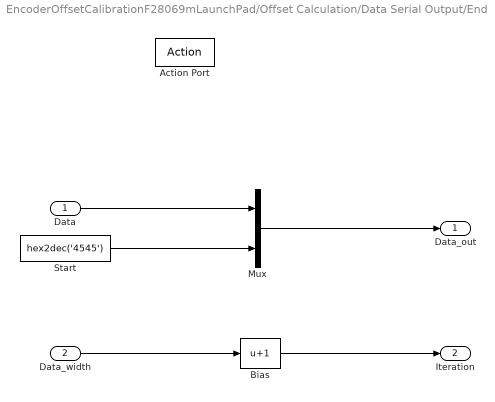
== system EncoderOffsetCalibrationF28069mLaunchPad/Offset Calculation/Data Serial Output/End ==
  Data : Inport
  Data_width : Inport  Port=2
  Action Port : ActionPort  ActionPortLabel=elseif(u1 == 599)
  Bias : Bias  Bias=1  SaturateOnIntegerOverflow=off
  Mux : Mux  Inputs=2
  Start : Constant  Value=hex2dec('4545')  OutDataTypeStr=uint16
  Data_out : Outport  VectorParamsAs1DForOutWhenUnconnected=off
  Iteration : Outport  Port=2  VectorParamsAs1DForOutWhenUnconnected=off
  wires:
  Mux/1 -> Data_out/1
  Data_width/1 -> Bias/1
  Start/1 -> Mux/2
  Bias/1 -> Iteration/1
  Data/1 -> Mux/1

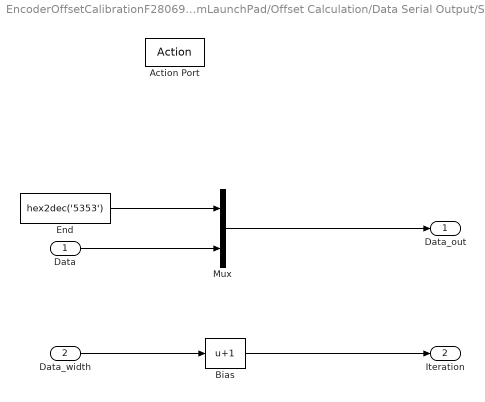
== system EncoderOffsetCalibrationF28069mLaunchPad/Offset Calculation/Data Serial Output/Start ==
  Data : Inport
  Data_width : Inport  Port=2
  Action Port : ActionPort  ActionPortLabel=if(u1 == 0)
  Bias : Bias  Bias=1  SaturateOnIntegerOverflow=off
  End : Constant  Value=hex2dec('5353')  OutDataTypeStr=uint16
  Mux : Mux  Inputs=2
  Data_out : Outport  VectorParamsAs1DForOutWhenUnconnected=off
  Iteration : Outport  Port=2  VectorParamsAs1DForOutWhenUnconnected=off
  wires:
  End/1 -> Mux/1
  Mux/1 -> Data_out/1
  Data_width/1 -> Bias/1
  Bias/1 -> Iteration/1
  Data/1 -> Mux/2

== system EncoderOffsetCalibrationF28069mLaunchPad/Offset Calculation/Data Serial Output/While Iterator Subsystem ==
  Data : Inport
  Iteration : Inport  Port=2
  Add : Sum  Inputs=+-  OutDataTypeStr=Inherit: Same as first input
  Index Vector : MultiPortSwitch  Inputs=1  SaturateOnIntegerOverflow=off  InputSameDT=off
  SCI Transmit : c280xlib/SCI Transmit  sciModule=A  dataHead=''  dataTail=''  frameSize=1  blockingMode=on  outputStatus=off
  While Iterator : WhileIterator  MaxIters=-1  WhileBlockType=do-while  ShowIterationPort=on  OutputDataType=int16
  wires:
  Iteration/1 -> Add/1
  Add/1 -> While Iterator/1
  Index Vector/1 -> SCI Transmit/1
  Data/1 -> Index Vector/2
  While Iterator/1 -> Index Vector/1, Add/2

== system EncoderOffsetCalibrationF28069mLaunchPad/Offset Calculation/Subsystem/Calculate Position from QEP count  ==
  Count : Inport
  Index : Inport  Port=2
  eQEP_Decoder : Subsystem
  Theta_e : Outport  InitialOutput=0  VectorParamsAs1DForOutWhenUnconnected=off
  wires:
  Index/1 -> eQEP_Decoder/2(Index)
  Count/1 -> eQEP_Decoder/1(Count)
  eQEP_Decoder/1(Theta_e) -> Theta_e/1

== system EncoderOffsetCalibrationF28069mLaunchPad/Offset Calculation/Control_System/PosGen/Subsystem ==
  Enable : EnablePort
  Constant : Constant  Value=0  OutDataTypeStr=Inherit: Inherit via back propagation
  Data Store Write : DataStoreWrite  DataStoreName=Enable  IndexOptions=Index vector (dialog)  Indices=1  OutputSizes=1
  wires:
  Constant/1 -> Data Store Write/1

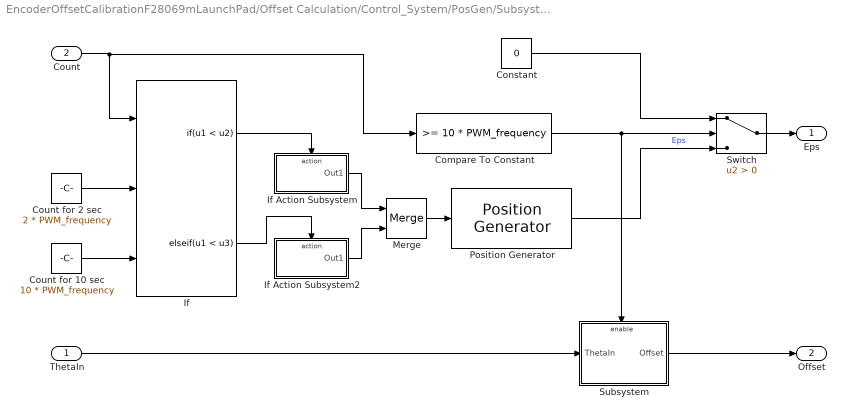
== system EncoderOffsetCalibrationF28069mLaunchPad/Offset Calculation/Control_System/PosGen/Subsystem1 ==
  ThetaIn : Inport
  Count : Inport  Port=2
  Compare To Constant : simulink/Logic and Bit Operations/Compare To Constant  relop=>=  const=10 * PWM_frequency  OutDataTypeStr=boolean
  Constant : Constant  Value=0  OutDataTypeStr=dataType  SampleTime=-1
  Count for 10 sec : Constant  Value=10 * PWM_frequency  OutDataTypeStr=uint32  SampleTime=-1
  Count for 2 sec : Constant  Value=2 * PWM_frequency  OutDataTypeStr=uint32  SampleTime=-1
  If : If  NumInputs=3  IfExpression=u1 < u2  ElseIfExpressions=u1 < u3  ShowElse=off
  If Action Subsystem : Subsystem  TreatAsAtomicUnit=on
  If Action Subsystem2 : Subsystem  TreatAsAtomicUnit=on
  Merge : Merge
  Position Generator : mcbcontrolslib/Position Generator  AngleOutput=Per-unit  InitialThetaSource=Specify via dialog  ExternalReset=none  Offset=0
  Subsystem : Subsystem
  Switch : Switch  Criteria=u2 > Threshold  SaturateOnIntegerOverflow=off  InputSameDT=off
  Eps : Outport
  Offset : Outport  Port=2
  wires:
  If Action Subsystem/1(Out1) -> Merge/1
  If/1 -> If Action Subsystem/Action
  If Action Subsystem2/1(Out1) -> Merge/2
  Count/1 -> Compare To Constant/1, If/1
  If/2 -> If Action Subsystem2/Action
  Merge/1 -> Position Generator/1
  Subsystem/1(Offset) -> Offset/1
  ThetaIn/1 -> Subsystem/1(ThetaIn)
  Switch/1 -> Eps/1
  Constant/1 -> Switch/1
  Position Generator/1 -> Switch/3  "Eps"
  Compare To Constant/1 -> Switch/2, Subsystem/Enable
  Count for 2 sec/1 -> If/2
  Count for 10 sec/1 -> If/3

== system EncoderOffsetCalibrationF28069mLaunchPad/Offset Calculation/Control_System/PosGen/Up counter ==
  Enable : EnablePort  StatesWhenEnabling=reset
  Add1 : Sum  SaturateOnIntegerOverflow=on
  Constant : Constant  OutDataTypeStr=uint32
  Delay : Delay  DelayLength=1
  Count : Outport  OutputWhenDisabled=reset  InitialOutput=0
  wires:
  Add1/1 -> Count/1, Delay/1
  Constant/1 -> Add1/1
  Delay/1 -> Add1/2

== system EncoderOffsetCalibrationF28069mLaunchPad/Offset Calculation/Subsystem/Calculate Position from QEP count /eQEP_Decoder ==
  Count : Inport
  Index : Inport  Port=2
  Mechanical to Electrical Position : mcbpositiondecoderlib/Mechanical to Electrical Position  PolePairsInputType=Specify via dialog  NrPP=motor.polePairs  selectedRange=Per unit  MechOfstInputType=Specify via dialog  mechOffsetIn=0  maxAngleIn=1  InputDataType=dataType  VariantSelect=floating-point
  Quadrature Decoder : mcbpositiondecoderlib/Quadrature Decoder  ParameterInputType=off  CountsPerRevInverseDataType=single  EncoderSlitsPerRevolution=motor.QEPSlits  EncoderCountsPerSlit=4  CounterSize=16 bits  ExternalIndexCount=on  PositionUnit=Per unit  PositionDataType=dataType
  Theta_e : Outport  VectorParamsAs1DForOutWhenUnconnected=off
  wires:
  Count/1 -> Quadrature Decoder/1
  Index/1 -> Quadrature Decoder/2
  Mechanical to Electrical Position/1 -> Theta_e/1
  Quadrature Decoder/1 -> Mechanical to Electrical Position/1

== system EncoderOffsetCalibrationF28069mLaunchPad/Offset Calculation/Control_System/PosGen/Subsystem1/If Action Subsystem ==
  Action Port : ActionPort  ActionPortLabel=if(u1 < u2)
  Constant : Constant  Value=0  OutDataTypeStr=dataType  SampleTime=-1
  Out1 : Outport
  wires:
  Constant/1 -> Out1/1

== system EncoderOffsetCalibrationF28069mLaunchPad/Offset Calculation/Control_System/PosGen/Subsystem1/If Action Subsystem2 ==
  Action Port : ActionPort  ActionPortLabel=elseif(u1 < u3)
  Add1 : Sum
  Constant1 : Constant  Value=1e-3  OutDataTypeStr=dataType  SampleTime=-1
  Delay : Delay  DelayLength=1
  Multiply : Gain  Gain=Ts  OutDataTypeStr=Inherit: Same as input
  Saturate to 'motor.calibSpeed' RPM : Saturate  UpperLimit=motor.polePairs * motor.calibSpeed / 60  LowerLimit=0
  Out1 : Outport
  wires:
  Delay/1 -> Add1/2
  Constant1/1 -> Add1/1
  Add1/1 -> Saturate to 'motor.calibSpeed' RPM/1
  Saturate to 'motor.calibSpeed' RPM/1 -> Multiply/1, Delay/1
  Multiply/1 -> Out1/1

== system EncoderOffsetCalibrationF28069mLaunchPad/Offset Calculation/Control_System/PosGen/Subsystem1/Subsystem ==
  ThetaIn : Inport
  Enable : EnablePort
  Multiply : Gain  Gain=1 / motor.polePairs  OutDataTypeStr=Inherit: Same as input
  Offset : Outport
  wires:
  ThetaIn/1 -> Multiply/1
  Multiply/1 -> Offset/1

== matlab function EncoderOffsetCalibrationF28069mLaunchPad/Offset Calculation/Read_AS5047P ==
function [spi_raw, spi_elec_pu] = Read_AS5047P()
%#codegen
% SPI-A AS5047P read on GPIO16/17/18 with GPIO19 chip select.
persistent init_done
spi_raw = uint16(0);
if coder.target('Rtw')
    coder.cinclude('as5047p_spi.h');
    coder.cinclude('qep_spi_sync.h');
    if isempty(init_done)
        coder.ceval('as5047p_spi_init');
        init_done = true;
    end
    coder.ceval('as5047p_spi_read', coder.ref(spi_raw));
    coder.ceval('seed_qep_from_spi', spi_raw);
end
spi_mech = single(spi_raw) * single(1.0 / 16384.0);
spi_elec_pu = mod(spi_mech * single(21.0), single(1.0));
end
